simulink model "model_wahadla_stribeck"  (R2023a)
settings: Solver=ode45  StartTime=0.0  StopTime=end_time  FixedStep=dt  MaxStep=0.001  RelTol=1e-3
values from neighbouring files (symbols this model uses):
  IC = [0;pi;0;0]    [system_id_2.m]
settings Model: Creator=Adam  LastModifiedBy=Adam
settings SolverCC: AlgebraicLoopSolver=TrustRegion
settings DataIOCC: ExternalInput=ind  LoadExternalInput=on  SignalLogging=off  DSMLogging=off  OutputSaveName=out  ReturnWorkspaceOutputsName=sout
settings DebuggingCC: AlgebraicLoopMsg=none  UnconnectedInputMsg=warning  UnconnectedOutputMsg=warning  UnconnectedLineMsg=warning
settings ModelReferenceCC: EnableRefExpFcnMdlSchedulingChecks=on
settings RTWCC: DLArmComputeVersion=19.05

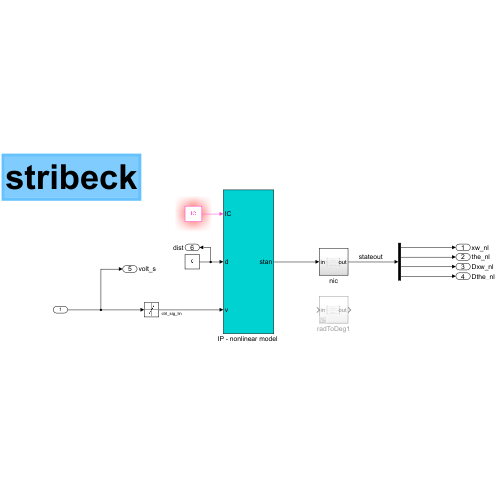
[thumbnail: Simulink's stored preview of the top-level diagram]
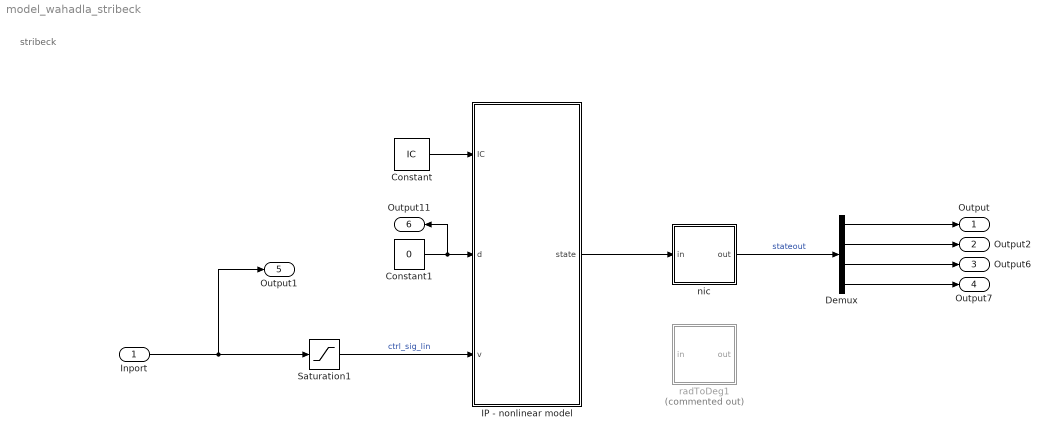
== system model_wahadla_stribeck ==
  note: stribeck
  Inport : Inport
  Constant : Constant  Value=IC  VectorParams1D=off
  Constant1 : Constant  Value=0
  Demux : Demux
  "IP - nonlinear model " : Subsystem  Description=Nonlinear model of inverted pendulum
      mask Display:
      | port_label('output', 1, 'stan');
      | port_label('input', 1, 'IC');
      | port_label('input', 2, 'd');
      | port_label('input', 3, 'v');
  Saturation1 : Saturate  UpperLimit=12  LowerLimit=-12
  nic : Subsystem
  radToDeg1 : Subsystem  Commented=on
  Output : Outport  SignalName=xw_nl
  Output2 : Outport  Port=2  SignalName=the_nl
  Output6 : Outport  Port=3  SignalName=Dxw_nl
  Output7 : Outport  Port=4  SignalName=Dthe_nl
  Output1 : Outport  Port=5  SignalName=volt_s
  Output11 : Outport  Port=6  SignalName=dist
  wires:
  Inport/1 -> Saturation1/1, Output1/1
  Constant1/1 -> "IP - nonlinear model "/2(d), Output11/1
  Saturation1/1 -> "IP - nonlinear model "/3(v)  "ctrl_sig_lin"
  Constant/1 -> "IP - nonlinear model "/1(IC)
  Demux/2 -> Output2/1
  nic/1(out) -> Demux/1  "stateout"
  "IP - nonlinear model "/1(state) -> nic/1(in)
  Demux/3 -> Output6/1
  Demux/1 -> Output/1
  Demux/4 -> Output7/1

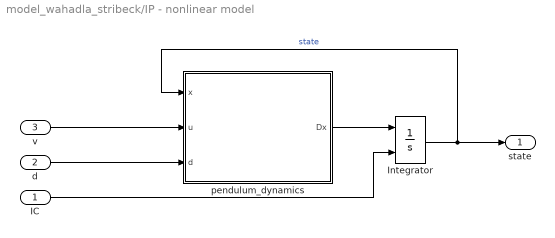
== system model_wahadla_stribeck/IP - nonlinear model  ==
  IC : Inport
  d : Inport  Port=2
  v : Inport  Port=3
  Integrator : Integrator  InitialConditionSource=external
  pendulum_dynamics : MATLAB Function  TreatAsAtomicUnit=on
  state : Outport
  wires:
  Integrator/1 -> state/1, pendulum_dynamics/1(x)  "state"
  v/1 -> pendulum_dynamics/2(u)
  pendulum_dynamics/1(Dx) -> Integrator/1
  IC/1 -> Integrator/2
  d/1 -> pendulum_dynamics/3(d)

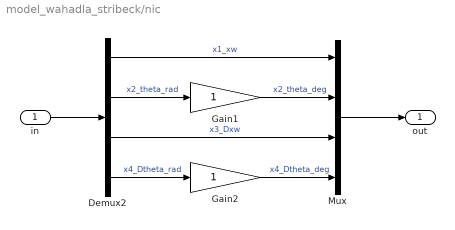
== system model_wahadla_stribeck/nic ==
  in : Inport
  Demux2 : Demux
  Gain1 : Gain
  Gain2 : Gain
  Mux : Mux
  out : Outport
  wires:
  Demux2/1 -> Mux/1  "x1_xw"
  Gain1/1 -> Mux/2  "x2_theta_deg"
  Gain2/1 -> Mux/4  "x4_Dtheta_deg"
  Demux2/2 -> Gain1/1  "x2_theta_rad"
  in/1 -> Demux2/1
  Demux2/3 -> Mux/3  "x3_Dxw"
  Demux2/4 -> Gain2/1  "x4_Dtheta_rad"
  Mux/1 -> out/1

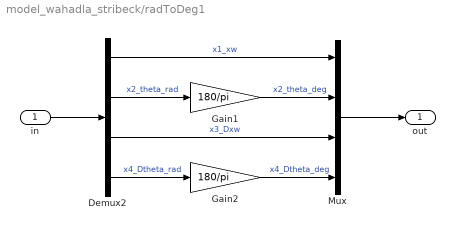
== system model_wahadla_stribeck/radToDeg1 ==
  in : Inport
  Demux2 : Demux
  Gain1 : Gain  Gain=180/pi
  Gain2 : Gain  Gain=180/pi
  Mux : Mux
  out : Outport
  wires:
  Demux2/1 -> Mux/1  "x1_xw"
  Gain1/1 -> Mux/2  "x2_theta_deg"
  Gain2/1 -> Mux/4  "x4_Dtheta_deg"
  Demux2/2 -> Gain1/1  "x2_theta_rad"
  in/1 -> Demux2/1
  Demux2/3 -> Mux/3  "x3_Dxw"
  Demux2/4 -> Gain2/1  "x4_Dtheta_rad"
  Mux/1 -> out/1

== matlab function model_wahadla_stribeck/IP - nonlinear model /pendulum_dynamics ==
  data: x input; u input; d input; Dx output; params_stribeck parameter
function Dx = dynamika_wahadla(x, u, d, params_stribeck)
% x : stan
% u : input - napięcie
%
% params scope: "parameters"
% State, function input: x = [x Dx theta Dtheta]'
    % x1 = x(1);
    x2 = x(2);
    x3 = x(3);
    x4 = x(4);
    params_stribeck = num2cell(params_stribeck);
    [M, mp, mc, Lp, alpha_dcm, B, gamma_stri, miu_c, miu_s, vs] = params_stribeck{:};
    g               = 9.8145;
    i_i             = 2;
    delta_          = 600;
    Lc = 2*Lp;
    mr = mc + mp;
    Mt = mr + M;
    L = (Lc*mc + Lp*mp) / mr;
    Jcm = 1/12*mp*Lp;
    Jt = Jcm + mr*L^2;
    
    % Ff = (miu_c + (miu_s-miu_c)*exp(-(x3/vs)^i_i)) * Mt*g*tanh(delta_*x3) + b_stri*x3;
    % Fi = alpha_dcm*u - beta_dcm*x3;
    Ff = (miu_c + (miu_s-miu_c)*exp(-(x3/vs)^i_i)) * Mt*g*tanh(delta_*x3);
    Fi = alpha_dcm*u;
    A = d*cos(x2) - Ff + L*mr*x4^2*sin(x2) + Fi - B*x3;
    B = d*Lc + L*g*mr*sin(x2) - gamma_stri*x4;
    DEN = Jt*Mt - (L*mr*cos(x2))^2;
    
    ddt_x1 = x3;
    ddt_x2 = x4;
    ddt_x3 = (Jt*A - L*mr*cos(x2)*B) / DEN;
    ddt_x4 = (Mt*B - L*mr*cos(x2)*A) / DEN;
    
    % output
    Dx = [ddt_x1 ddt_x2 ddt_x3 ddt_x4]';
end
